simulink model "spike_detection_model"  (R2018b)
settings: Solver=VariableStepAuto  StartTime=0.0  StopTime=50000  RelTol=1e-3
settings Model: Creator=diyar  LastModifiedBy=diyar
settings DataIOCC: ExternalInput=shaped.getElement('shaped_data')

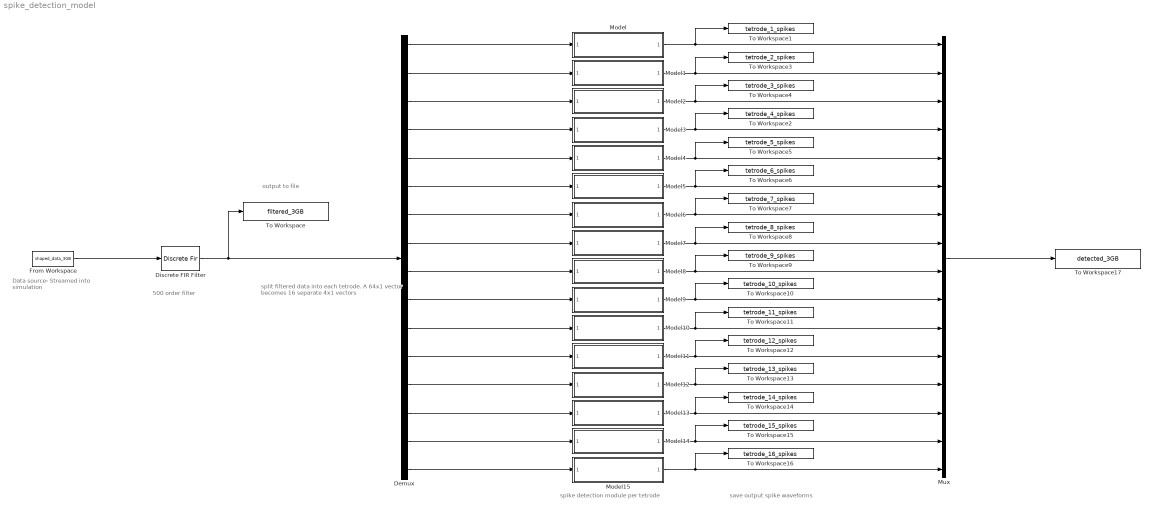
== system spike_detection_model ==
  note: save output spike waveforms
  note: spike detection module per tetrode
  note: output to file
  note: Data source- Streamed into simulation
  note: split filtered data into each tetrode. A 64x1 vector becomes 16 separate 4x1 vectors
  note: 500 order filter
  Demux : Demux  Outputs=16
  Discrete FIR Filter : DiscreteFir  Coefficients="[-8.17821769629145e-05\t1.52360144582896e-05\t6.67989529459943e-05\t1.45982532170905e-05\t-9.82482226870618e-05\t-0.000167720088805530\t-0.000130359932843811\t-2.69992057115584e-05\t3.50481496681095e-05\t-1.34222581784301e-05\t-0.000133737349284299\t-0.000214476507917817\t-0.000179890380891333\t-6.64167473462355e-05\t9.74546177215107e-06\t-3.44149869897154e-05\t-0.000164678527290800\t-0.000259215332805959\t-0.000226764643636769\t-9.90566838800375e-05\t-4.17771720731235e-06\t-4.24686961314622e-05\t-0.000184802469867880\t-0.000295970779758922\t-0.000265385769419656\t-0.000119096341177723\t-1.60688080874614e-18\t-2.98847804617079e-05\t-0.000186060443838235\t-0.000317107102327633\t-0.000288721594028980\t-0.000119565212930064\t2.99070260133799e-05\t1.17777156253048e-05\t-0.000159819004971979\t-0.000314654974790004\t-0.000289784140566015\t-9.39729213581581e-05\t9.23031015468184e-05\t8.97914039647651e-05\t-9.88858712022507e-05\t-0.000282436135327971\t-0.000263845972053216\t-3.86152492758540e-05\t0.000190690844858293\t0.000207808301849631\t-1.30174564005612e-19\t-0.000218568189321096\t-0.000210946022572317\t4.49266986883817e-05\t0.000322834792433222\t0.000363418972241649\t0.000133796719011513\t-0.000127740704264635\t-0.000138053204796511\t0.000147745289076766\t0.000478854810992852\t0.000546401817619709\t0.000291592496484421\t-2.25732125004858e-05\t-6.01998709803687e-05\t0.000252705225011073\t0.000640565903784929\t0.000738319990763398\t0.000454481561552431\t7.65588683781077e-05\t-3.15660171913448e-18\t0.000335234419882821\t0.000782579100074059\t0.000913939315949503\t0.000597310859866505\t0.000143608568227651\t1.47724366892927e-05\t0.000366074474447542\t0.000875371240697318\t0.00104461260066473\t0.000692377770534116\t0.000150864389856078\t-4.45126497680444e-05\t0.000315861693227001\t0.000890122344319080\t0.00110335631624446\t0.000714731638118502\t7.44592137383561e-05\t-0.000201649711273897\t0.000160971680822901\t0.000804682797132406\t0.00107091327065005\t0.000648306226876088\t-9.94562760235953e-05\t-0.000469417247096643\t-0.000110330293148178\t0.000609658470944248\t0.000941740071186134\t0.000491777127174730\t-0.000369022114246030\t-0.000844091300800617\t-0.000492645867129614\t0.000313377293397299\t0.000728665975274091\t0.000262880116493016\t-0.000712728401375181\t-0.00130192068969815\t-0.000960367268965271\t-5.55073304596875e-05\t0.000465002059893442\t-7.87060208769412e-18\t-0.00108837936392093\t-0.00179867543640600\t-0.00146783036000224\t-0.000448781388768246\t0.000203160560670888\t-0.000239838720692055\t-0.00143575442289967\t-0.00227297993901411\t-0.00195332237594296\t-0.000803335819804737\t9.35152888739072e-06\t-0.000386908008287064\t-0.00168318841263872\t-0.00265354494320378\t-0.00234694749004362\t-0.00104962038521951\t-4.54109412907271e-05\t-0.000368285380848779\t-0.00175759680047743\t-0.00286970634166996\t-0.00258164100772558\t-0.00112305761689692\t0.000102956145809872\t-0.000119867727708134\t-0.00159676444752790\t-0.00286398324351772\t-0.00260594295977811\t-0.000976926661168878\t0.000498718790705944\t0.000400796175644003\t-0.00116212715051938\t-0.00260481200115535\t-0.00239662318905965\t-0.000594746816662970\t0.00115432032282929\t0.00120293861516712\t-0.000449923973831185\t-0.00209731354589300\t-0.00196900526674699\t1.59245520223221e-18\t0.00204142453276093\t0.00225443904831509\t0.000501426662407912\t-0.00138998979874324\t-0.00138293987461840\t0.000738803764086166\t0.00308695441968850\t0.00347901321576363\t0.00160953571159591\t-0.000575649542595459\t-0.000742849153621883\t0.00150918403160290\t0.00417549426914411\t0.00475998976650475\t0.00275296827457575\t0.000214398697577091\t-0.000191059605913733\t0.00216249505455281\t0.00515855129592762\t0.00595104364997675\t0.00378308708565251\t0.000822873976247832\t0.000105337801291035\t0.00252805705263439\t0.00587013012653614\t0.00689322390182507\t0.00454197910005902\t0.00108468734634293\t-2.72417575153595e-05\t0.00243209065724959\t0.00614701863040120\t0.00743661866396499\t0.00488465940365572\t0.000848664898609861\t-0.000747844968971962\t0.00171893162502487\t0.00585129043408973\t0.00746423454606267\t0.00470303810378778\t3.79532254589281e-18\t-0.00218036907074136\t0.000271235377232089\t0.00489195613648307\t0.00691532575076598\t0.00394888392305232\t-0.00151976117072625\t-0.00439708259678841\t-0.00197460310079623\t0.00324255718160911\t0.00580569421070923\t0.00265343177046898\t-0.00369829345677855\t-0.00741031387611637\t-0.00502190436425862\t0.000951844301734861\t0.00424367773962046\t0.000942673125399890\t-0.00644613234468655\t-0.0111768603992220\t-0.00882075718487963\t-0.00185450920140287\t0.00244327772568692\t-0.000949516397838462\t-0.00959988089811970\t-0.0156216094635979\t-0.0132958169569060\t-0.00498204163175538\t0.000742082385076925\t-0.00266104708044969\t-0.0129351968663042\t-0.0206941294194402\t-0.0184110305836446\t-0.00818500388056339\t-0.000351622648878286\t-0.00364450702418185\t-0.0161883865286444\t-0.0264993588781159\t-0.0243219413397020\t-0.0111913896165012\t3.41858951050374e-18\t-0.00297006011540962\t-0.0190841568363699\t-0.0336623603377464\t-0.0318218584570029\t-0.0137325141454559\t0.00359461010710019\t0.00148868352108431\t-0.0213661123547914\t-0.0447957449568108\t-0.0442910228991483\t-0.0155734135851870\t0.0167909324332271\t0.0182120296537261\t-0.0228260844534596\t-0.0763105004360396\t-0.0869108081892783\t-0.0165401077222937\t0.119478683408986\t0.253933304568958\t0.309934916210110\t0.253933304568958\t0.119478683408986\t-0.0165401077222937\t-0.0869108081892783\t-0.0763105004360396\t-0.0228260844534596\t0.0182120296537261\t0.0167909324332271\t-0.0155734135851870\t-0.0442910228991483\t-0.0447957449568108\t-0.0213661123547914\t0.00148868352108431\t0.00359461010710019\t-0.0137325141454559\t-0.0318218584570029\t-0.0336623603377464\t-0.0190841568363699\t-0.00297006011540962\t3.41858951050374e-18\t-0.0111913896165012\t-0.0243219413397020\t-0.0264993588781159\t-0.0161883865286444\t-0.00364450702418185\t-0.000351622648878286\t-0.00818500388056339\t-0.0184110305836446\t-0.0206941294194402\t-0.0129351968663042\t-0.00266104708044969\t0.000742082385076925\t-0.00498204163175538\t-0.0132958169569060\t-0.0156216094635979\t-0.00959988089811970\t-0.000949516397838462\t0.00244327772568692\t-0.00185450920140287\t-0.00882075718487963\t-0.0111768603992220\t-0.00644613234468655\t0.000942673125399890\t0.00424367773962046\t0.000951844301734861\t-0.00502190436425862\t-0.00741031387611637\t-0.00369829345677855\t0.00265343177046898\t0.00580569421070923\t0.00324255718160911\t-0.00197460310079623\t-0.00439708259678841\t-0.00151976117072625\t0.00394888392305232\t0.00691532575076598\t0.00489195613648307\t0.000271235377232089\t-0.00218036907074136\t3.79532254589281e-18\t0.00470303810378778\t0.00746423454606267\t0.00585129043408973\t0.00171893162502487\t-0.000747844968971962\t0.000848664898609861\t0.00488465940365572\t0.00743661866396499\t0.00614701863040120\t0.00243209065724959\t-2.72417575153595e-05\t0.00108468734634293\t0.00454197910005902\t0.00689322390182507\t0.00587013012653614\t0.00252805705263439\t0.000105337801291035\t0.000822873976247832\t0.00378308708565251\t0.00595104364997675\t0.00515855129592762\t0.00216249505455281\t-0.000191059605913733\t0.000214398697577091\t0.00275296827457575\t0.00475998976650475\t0.00417549426914411\t0.00150918403160290\t-0.000742849153621883\t-0.000575649542595459\t0.00160953571159591\t0.00347901321576363\t0.00308695441968850\t0.000738803764086166\t-0.00138293987461840\t-0.00138998979874324\t0.000501426662407912\t0.00225443904831509\t0.00204142453276093\t1.59245520223221e-18\t-0.00196900526674699\t-0.00209731354589300\t-0.000449923973831185\t0.00120293861516712\t0.00115432032282929\t-0.000594746816662970\t-0.00239662318905965\t-0.00260481200115535\t-0.00116212715051938\t0.000400796175644003\t0.000498718790705944\t-0.000976926661168878\t-0.00260594295977811\t-0.00286398324351772\t-0.00159676444752790\t-0.000119867727708134\t0.000102956145809872\t-0.00112305761689692\t-0.00258164100772558\t-0.00286970634166996\t-0.00175759680047743\t-0.000368285380848779\t-4.54109412907271e-05\t-0.00104962038521951\t-0.00234694749004362\t-0.00265354494320378\t-0.00168318841263872\t-0.000386908008287064\t9.35152888739072e-06\t-0.000803335819804737\t-0.00195332237594296\t-0.00227297993901411\t-0.00143575442289967\t-0.000239838720692055\t0.000203160560670888\t-0.000448781388768246\t-0.00146783036000224\t-0.00179867543640600\t-0.00108837936392093\t-7.87060208769412e-18\t0.000465002059893442\t-5.55073304596875e-05\t-0.000960367268965271\t-0.00130192068969815\t-0.000712728401375181\t0.000262880116493016\t0.000728665975274091\t0.000313377293397299\t-0.000492645867129614\t-0.000844091300800617\t-0.000369022114246030\t0.000491777127174730\t0.000941740071186134\t0.000609658470944248\t-0.000110330293148178\t-0.000469417247096643\t-9.94562760235953e-05\t0.000648306226876088\t0.00107091327065005\t0.000804682797132406\t0.000160971680822901\t-0.000201649711273897\t7.44592137383561e-05\t0.000714731638118502\t0.00110335631624446\t0.000890122344319080\t0.000315861693227001\t-4.45126497680444e-05\t0.000150864389856078\t0.000692377770534116\t0.00104461260066473\t0.000875371240697318\t0.000366074474447542\t1.47724366892927e-05\t0.000143608568227651\t0.000597310859866505\t0.000913939315949503\t0.000782579100074059\t0.000335234419882821\t-3.15660171913448e-18\t7.65588683781077e-05\t0.000454481561552431\t0.000738319990763398\t0.000640565903784929\t0.000252705225011073\t-6.01998709803687e-05\t-2.25732125004858e-05\t0.000291592496484421\t0.000546401817619709\t0.000478854810992852\t0.000147745289076766\t-0.000138053204796511\t-0.000127740704264635\t0.000133796719011513\t0.000363418972241649\t0.000322834792433222\t4.49266986883817e-05\t-0.000210946022572317\t-0.000218568189321096\t-1.30174564005612e-19\t0.000207808301849631\t0.000190690844858293\t-3.86152492758540e-05\t-0.000263845972053216\t-0.000282436135327971\t-9.88858712022507e-05\t8.97914039647651e-05\t9.23031015468184e-05\t-9.39729213581581e-05\t-0.000289784140566015\t-0.000314654974790004\t-0.000159819004971979\t1.17777156253048e-05\t2.99070260133799e-05\t-0.000119565212930064\t-0.000288721594028980\t-0.000317107102327633\t-0.000186060443838235\t-2.98847804617079e-05\t-1.60688080874614e-18\t-0.000119096341177723\t-0.000265385769419656\t-0.000295970779758922\t-0.000184802469867880\t-4.24686961314622e-05\t-4.17771720731235e-06\t-9.90566838800375e-05\t-0.000226764643636769\t-0.000259215332805959\t-0.000164678527290800\t-3.44149869897154e-05\t9.74546177215107e-06\t-6.64167473462355e-05\t-0.000179890380891333\t-0.000214476507917817\t-0.000133737349284299\t-1.34222581784301e-05\t3.50481496681095e-05\t-2.69992057115584e-05\t-0.000130359932843811\t-0.000167720088805530\t-9.82482226870618e-05\t1.45982532170905e-05\t6.67989529459943e-05\t1.52360144582896e-05\t-8.17821769629145e-05\t-0.000122837897653802\t-6.24361387451902e-05\t4.56484255495584e-05\t0.000101837778480746]"
  From Workspace : FromWorkspace  VariableName=shaped_data_3GB  SampleTime=1
  Model{,1..15} (16 alike) : ModelReference  ModelNameDialog=spike_detection  SimulationMode=Normal  ModelReferenceVersion=1.10
  Mux : Mux  Inputs=16
  To Workspace : ToWorkspace  VariableName=filtered_3GB  SampleTime=-1
      settings: Save2DSignal=2-D array (concatenate along first dimension)
  To Workspace1 : ToWorkspace  VariableName=tetrode_1_spikes  SaveFormat=Structure With Time  SampleTime=-1
  To Workspace10 : ToWorkspace  VariableName=tetrode_10_spikes  SaveFormat=Structure With Time  SampleTime=-1
  To Workspace11 : ToWorkspace  VariableName=tetrode_11_spikes  SaveFormat=Structure With Time  SampleTime=-1
  To Workspace12 : ToWorkspace  VariableName=tetrode_12_spikes  SaveFormat=Structure With Time  SampleTime=-1
  To Workspace13 : ToWorkspace  VariableName=tetrode_13_spikes  SaveFormat=Structure With Time  SampleTime=-1
  To Workspace14 : ToWorkspace  VariableName=tetrode_14_spikes  SaveFormat=Structure With Time  SampleTime=-1
  To Workspace15 : ToWorkspace  VariableName=tetrode_15_spikes  SaveFormat=Structure With Time  SampleTime=-1
  To Workspace16 : ToWorkspace  VariableName=tetrode_16_spikes  SaveFormat=Structure With Time  SampleTime=-1
  To Workspace17 : ToWorkspace  VariableName=detected_3GB  SampleTime=-1
      settings: Save2DSignal=2-D array (concatenate along first dimension)
  To Workspace2 : ToWorkspace  VariableName=tetrode_4_spikes  SaveFormat=Structure With Time  SampleTime=-1
  To Workspace3 : ToWorkspace  VariableName=tetrode_2_spikes  SaveFormat=Structure With Time  SampleTime=-1
  To Workspace4 : ToWorkspace  VariableName=tetrode_3_spikes  SaveFormat=Structure With Time  SampleTime=-1
  To Workspace5 : ToWorkspace  VariableName=tetrode_5_spikes  SaveFormat=Structure With Time  SampleTime=-1
  To Workspace6 : ToWorkspace  VariableName=tetrode_6_spikes  SaveFormat=Structure With Time  SampleTime=-1
  To Workspace7 : ToWorkspace  VariableName=tetrode_7_spikes  SaveFormat=Structure With Time  SampleTime=-1
  To Workspace8 : ToWorkspace  VariableName=tetrode_8_spikes  SaveFormat=Structure With Time  SampleTime=-1
  To Workspace9 : ToWorkspace  VariableName=tetrode_9_spikes  SaveFormat=Structure With Time  SampleTime=-1
  wires:
  Demux/1 -> Model/1
  Demux/2 -> Model1/1
  Demux/3 -> Model2/1
  Demux/4 -> Model3/1
  Demux/5 -> Model4/1
  Demux/6 -> Model5/1
  Demux/7 -> Model6/1
  Demux/8 -> Model7/1
  Demux/9 -> Model8/1
  Demux/10 -> Model9/1
  Demux/11 -> Model10/1
  Demux/12 -> Model11/1
  Demux/13 -> Model12/1
  Demux/14 -> Model13/1
  Demux/15 -> Model14/1
  Demux/16 -> Model15/1
  Model/1 -> Mux/1, To Workspace1/1
  Model1/1 -> Mux/2, To Workspace3/1
  Model3/1 -> Mux/4, To Workspace2/1
  Model4/1 -> Mux/5, To Workspace5/1
  Model5/1 -> Mux/6, To Workspace6/1
  Model6/1 -> Mux/7, To Workspace7/1
  Model8/1 -> Mux/9, To Workspace9/1
  Model9/1 -> Mux/10, To Workspace10/1
  Model10/1 -> Mux/11, To Workspace11/1
  Model11/1 -> Mux/12, To Workspace12/1
  Model12/1 -> Mux/13, To Workspace13/1
  Model13/1 -> Mux/14, To Workspace14/1
  Model14/1 -> Mux/15, To Workspace15/1
  Model7/1 -> Mux/8, To Workspace8/1
  Model2/1 -> Mux/3, To Workspace4/1
  Model15/1 -> Mux/16, To Workspace16/1
  Mux/1 -> To Workspace17/1
  From Workspace/1 -> Discrete FIR Filter/1
  Discrete FIR Filter/1 -> To Workspace/1, Demux/1
